simulink model "L0704_1"  (Simulink 10.2)
settings: Solver=ode45  StartTime=0.0  StopTime=10  MaxStep=0.01  RelTol=1e-3
InitFcn:
  | data
values from neighbouring files (symbols this model uses):
  g = 9.81    [data.m]
  Vx0 = 5    [data.m]
  Vy0 = 16    [data.m]
  x0 = []    [L0706Plot.m]    (also in L0708Plot.m; data.m = 1)
  y0 = 5    [data.m]
libraries: simulink x2
settings Model: Creator=Ranci  LastModifiedBy=Ranci
settings DataIOCC: SaveFormat=Dataset  SignalLoggingSaveFormat=Dataset  ReturnWorkspaceOutputs=on
settings OptimizationCC: LifeSpan=auto
settings DebuggingCC: UnderspecifiedInitializationDetection=Simplified  MergeDetectMultiDrivingBlocksExec=error  FcnCallInpInsideContextMsg=error  SFUnexpectedBacktrackingDiag=error  SFNoUnconditionalDefaultTransitionDiag=error  SFExecutionAtInitializationDiag=warning  ArithmeticOperatorsInVariantConditions=error
settings HardwareCC: ProdBitPerPointer=64  ProdBitPerSizeT=64  ProdBitPerPtrDiffT=64  ProdLargestAtomicFloat=Float  ProdIntDivRoundTo=Zero  ProdEndianess=LittleEndian  ProdWordSize=64  ProdHWDeviceType=Intel->x86-64 (Windows64)
settings ModelReferenceCC: PropagateSignalLabelsOutOfModel=on
settings SFSimCC: SimUseLocalCustomCode=on  CustomCodeUndefinedFunction=FilterOut
settings RTWCC: RTWUseLocalCustomCode=on
settings CodeAppCC: StateflowObjectComments=off
settings GRTTargetCC: TargetLangStandard=C99 (ISO)  CombineOutputUpdateFcns=on  GRTInterface=off
settings ConfigComp: CovMetricSettings=dwe  CovSaveCumulativeToWorkspaceVar=off  CovSaveSingleToWorkspaceVar=off  CovExternalEMLEnable=on

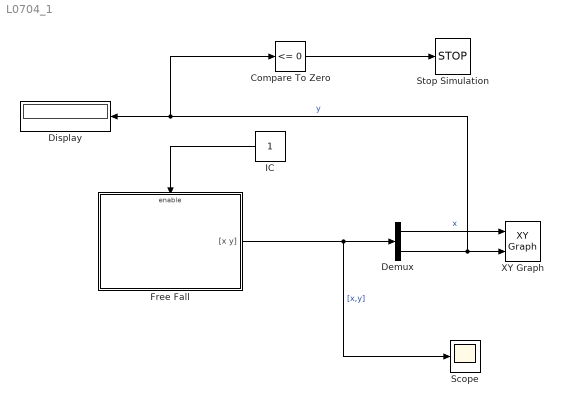
== system L0704_1 ==
  Compare To Zero : simulink/Logic and Bit Operations/Compare To Zero  relop=<=  OutDataTypeStr=boolean
  Demux : Demux  Outputs=2
  Display : Display
  Free Fall : Subsystem  TreatAsAtomicUnit=on
  IC : Constant
  Scope : Scope
  Stop Simulation : Stop
  XY Graph : simulink/Sinks/XY Graph  xmin=0  xmax=20  ymin=0  ymax=20  st=-1
  wires:
  Free Fall/1("[x y]") -> Scope/1, Demux/1  "[x,y]"
  Demux/1 -> XY Graph/1  "x"
  Demux/2 -> Compare To Zero/1, Display/1, XY Graph/2  "y"
  Compare To Zero/1 -> Stop Simulation/1
  IC/1 -> Free Fall/Enable

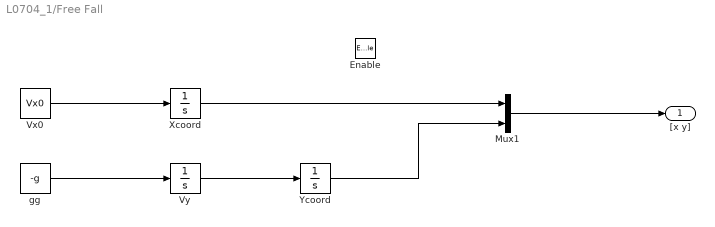
== system L0704_1/Free Fall ==
  Enable : EnablePort
  Mux1 : Mux  Inputs=2
  Vx0 : Constant  Value=Vx0
  Vy : Integrator  InitialCondition=Vy0
  Xcoord : Integrator  InitialCondition=x0
  Ycoord : Integrator  InitialCondition=y0
  gg : Constant  Value=-g
  "[x y]" : Outport
  wires:
  Vx0/1 -> Xcoord/1
  gg/1 -> Vy/1
  Vy/1 -> Ycoord/1
  Xcoord/1 -> Mux1/1
  Ycoord/1 -> Mux1/2
  Mux1/1 -> "[x y]"/1
